simulink model "OSWEC_latching_force"  (R2021b)
settings: Solver=ode4  StartTime=0  StopTime=400  FixedStep=0.01  MaxStep=0.01  RelTol=1e-3  EnableMultiTasking=on
values from neighbouring files (symbols this model uses):
  simu = simulationClass()    [wecSimInputFile.m]
  waves = waveClass('regular')    [wecSimInputFile.m]
undefined symbols (not defined in the file or in its folder): body, constraint, geometry, hydroData, pto, X, Y, Z
libraries: nesl_utility x31, sm_lib x23, WECSim_Lib_Body_Elements x7, WECSim_Lib_Constraints x1, vrlib x1, WECSim_Lib_Frames x1
(part 3 of 3)

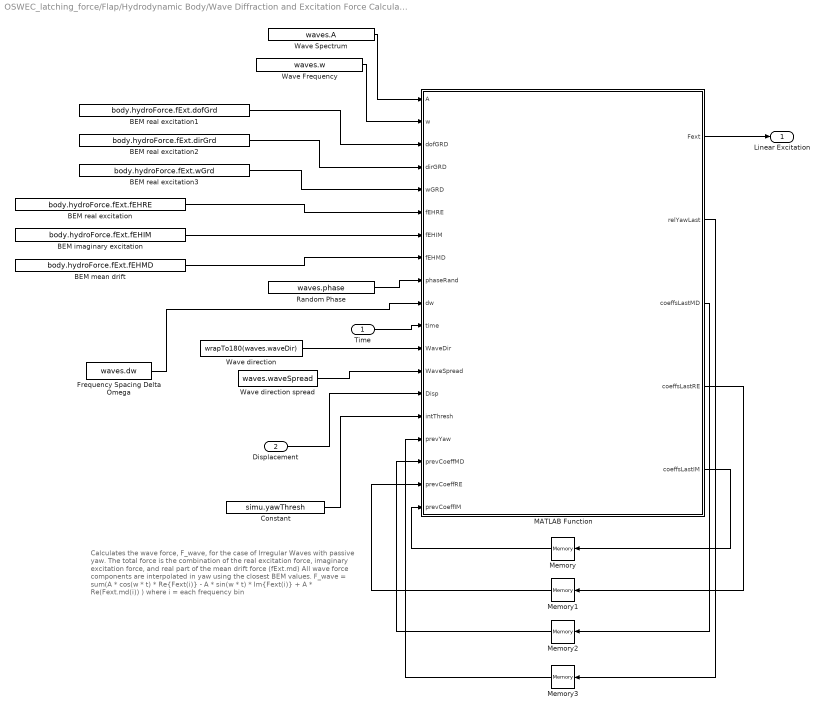
== system OSWEC_latching_force/Flap/Hydrodynamic Body/Wave Diffraction and Excitation Force Calculation/Linear Wave Excitation Force Variant Subsystem/Irregular Wave NonLinearYaw ==
  note: Calculates the wave force, F_wave, for the case of Irregular Waves with passive yaw.
      |
      | The total force is the combination of the real excitation force, imaginary excitation force, and real part of the mean drift force (fExt.md)
      |
      | All wave force components are interpolated in yaw using the closest BEM values.
      |
      | F_wave =   sum(A * cos(w * t) * Re{Fext(i)}
      |                            -  A * sin(w * t) * Im{Fext(i)}
      |                            + A * Re(Fext.md(i))
      |                            )
      |
      | where i = each frequency bin
  Time : Inport
  Displacement : Inport  Port=2
  BEM imaginary excitation : Constant  Value=body.hydroForce.fExt.fEHIM  VectorParams1D=off
  BEM mean drift : Constant  Value=body.hydroForce.fExt.fEHMD  VectorParams1D=off
  BEM real excitation : Constant  Value=body.hydroForce.fExt.fEHRE  VectorParams1D=off
  BEM real excitation1 : Constant  Value=body.hydroForce.fExt.dofGrd  VectorParams1D=off
  BEM real excitation2 : Constant  Value=body.hydroForce.fExt.dirGrd  VectorParams1D=off
  BEM real excitation3 : Constant  Value=body.hydroForce.fExt.wGrd  VectorParams1D=off
  Constant : Constant  Value=simu.yawThresh
  Frequency Spacing Delta Omega : Constant  Value=waves.dw  VectorParams1D=off
  MATLAB Function : MATLAB Function  TreatAsAtomicUnit=on
  Memory{,1..3} (4 alike) : Memory  InheritSampleTime=on  LinearizeAsDelay=on
  Random Phase : Constant  Value=waves.phase  VectorParams1D=off
  Wave Frequency : Constant  Value=waves.w  VectorParams1D=off
  Wave Spectrum : Constant  Value=waves.A  VectorParams1D=off
  Wave direction : Constant  Value=wrapTo180(waves.waveDir)  VectorParams1D=off
  Wave direction spread : Constant  Value=waves.waveSpread  VectorParams1D=off
  Linear Excitation : Outport
  wires:
  Displacement/1 -> MATLAB Function/14(Disp)
  Time/1 -> MATLAB Function/11(time)
  Wave direction spread/1 -> MATLAB Function/13(WaveSpread)
  BEM mean drift/1 -> MATLAB Function/8(fEHMD)
  Wave Spectrum/1 -> MATLAB Function/1(A)
  BEM real excitation1/1 -> MATLAB Function/3(dofGRD)
  Wave Frequency/1 -> MATLAB Function/2(w)
  Random Phase/1 -> MATLAB Function/9(phaseRand)
  Memory/1 -> MATLAB Function/19(prevCoeffIM)
  BEM real excitation/1 -> MATLAB Function/6(fEHRE)
  MATLAB Function/3(coeffsLastMD) -> Memory2/1
  Constant/1 -> MATLAB Function/15(intThresh)
  BEM imaginary excitation/1 -> MATLAB Function/7(fEHIM)
  Memory3/1 -> MATLAB Function/16(prevYaw)
  MATLAB Function/5(coeffsLastIM) -> Memory/1
  Wave direction/1 -> MATLAB Function/12(WaveDir)
  Frequency Spacing Delta Omega/1 -> MATLAB Function/10(dw)
  BEM real excitation2/1 -> MATLAB Function/4(dirGRD)
  BEM real excitation3/1 -> MATLAB Function/5(wGRD)
  Memory2/1 -> MATLAB Function/17(prevCoeffMD)
  MATLAB Function/2(relYawLast) -> Memory3/1
  MATLAB Function/4(coeffsLastRE) -> Memory1/1
  Memory1/1 -> MATLAB Function/18(prevCoeffRE)
  MATLAB Function/1(Fext) -> Linear Excitation/1

== system OSWEC_latching_force/Flap/Hydrodynamic Body/Wave Diffraction and Excitation Force Calculation/Linear Wave Excitation Force Variant Subsystem/No Wave Excitation Force ==
  Constant : Constant  Value=zeros(1,body.dof)
  Linear Excitation : Outport
  wires:
  Constant/1 -> Linear Excitation/1

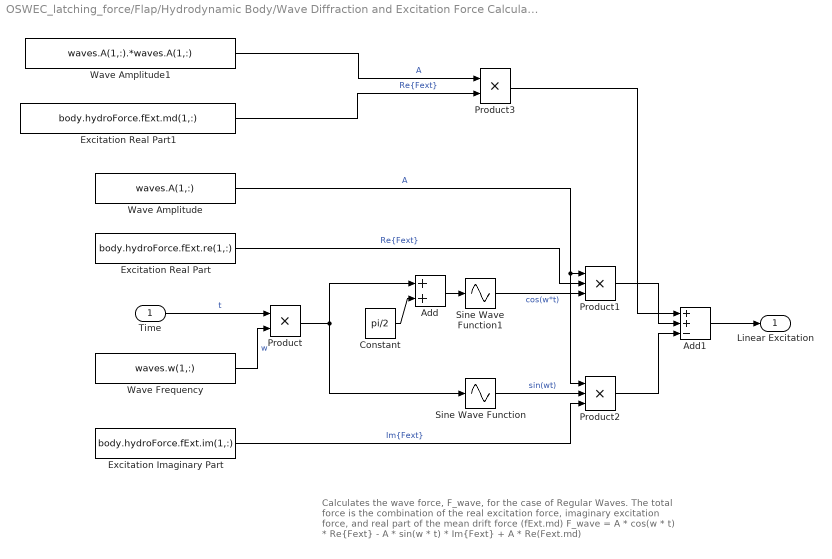
== system OSWEC_latching_force/Flap/Hydrodynamic Body/Wave Diffraction and Excitation Force Calculation/Linear Wave Excitation Force Variant Subsystem/Regular Wave Excitation Force ==
  note: Calculates the wave force, F_wave, for the case of Regular Waves.
      |
      | The total force is the combination of the real excitation force, imaginary excitation force, and real part of the mean drift force (fExt.md)
      |
      | F_wave =   A * cos(w * t) * Re{Fext}
      |                -  A * sin(w * t) * Im{Fext}
      |                + A * Re(Fext.md)
  Time : Inport
  Add : Sum
  Add1 : Sum  Inputs=++-
  Constant : Constant  Value=pi/2
  Excitation Imaginary Part : Constant  Value=body.hydroForce.fExt.im(1,:)  VectorParams1D=off
  Excitation Real Part : Constant  Value=body.hydroForce.fExt.re(1,:)  VectorParams1D=off
  Excitation Real Part1 : Constant  Value=body.hydroForce.fExt.md(1,:)  VectorParams1D=off
  Product : Product
  Product1 : Product  Inputs=3
  Product2 : Product  Inputs=3
  Product3 : Product
  Sine Wave Function : Sin  TimeSource=Use external signal  SampleTime=0
  Sine Wave Function1 : Sin  TimeSource=Use external signal  SampleTime=0
  Wave Amplitude : Constant  Value=waves.A(1,:)
  Wave Amplitude1 : Constant  Value=waves.A(1,:).*waves.A(1,:)
  Wave Frequency : Constant  Value=waves.w(1,:)
  Linear Excitation : Outport
  wires:
  Product3/1 -> Add1/1
  Excitation Real Part1/1 -> Product3/2  "Re{Fext}"
  Wave Amplitude1/1 -> Product3/1  "A"
  Constant/1 -> Add/2
  Add/1 -> Sine Wave Function1/1
  Wave Amplitude/1 -> Product1/1, Product2/1  "A"
  Add1/1 -> Linear Excitation/1
  Product2/1 -> Add1/3
  Product1/1 -> Add1/2
  Excitation Real Part/1 -> Product1/2  "Re{Fext}"
  Excitation Imaginary Part/1 -> Product2/3  "Im{Fext}"
  Sine Wave Function/1 -> Product2/2  "sin(wt)"
  Sine Wave Function1/1 -> Product1/3  "cos(w*t)"
  Product/1 -> Add/1, Sine Wave Function/1
  Wave Frequency/1 -> Product/2  "w"
  Time/1 -> Product/1  "t"

== system OSWEC_latching_force/Flap/Hydrodynamic Body/Wave Diffraction and Excitation Force Calculation/Linear Wave Excitation Force Variant Subsystem/Regular Wave NonLinear Yaw ==
  note: Calculates the wave force, F_wave, for the case of Regular Waves with passive yaw.
      |
      | The total force is the combination of the real excitation force, imaginary excitation force, and real part of the mean drift force (fExt.md)
      |
      | All wave force components are interpolated in yaw using the closest BEM values.
      |
      | F_wave =   A * cos(w * t) * Re{Fext}
      |                -  A * sin(w * t) * Im{Fext}
      |                + A * Re(Fext.md)
  Time : Inport
  Displacement : Inport  Port=2
  BEM imaginary excitation : Constant  Value=body.hydroForce.fExt.fEHIM  VectorParams1D=off
  BEM imaginary excitation1 : Constant  Value=body.hydroForce.fExt.dirGrd  VectorParams1D=off
  BEM mean drift : Constant  Value=body.hydroForce.fExt.fEHMD  VectorParams1D=off
  BEM real excitation : Constant  Value=body.hydroForce.fExt.fEHRE  VectorParams1D=off
  BEM real excitation1 : Constant  Value=body.hydroForce.fExt.dofGrd  VectorParams1D=off
  Constant : Constant  Value=simu.yawThresh
  MATLAB Function1 : MATLAB Function  TreatAsAtomicUnit=on
  Memory{,1..3} (4 alike) : Memory  InheritSampleTime=on  LinearizeAsDelay=on
  Wave Amplitude : Constant  Value=waves.A(1,:)
  Wave Frequency : Constant  Value=waves.w(1,:)
  Wave direction : Constant  Value=wrapTo180(waves.waveDir)  VectorParams1D=off
  Linear Excitation : Outport
  wires:
  Displacement/1 -> MATLAB Function1/10(Disp)
  Time/1 -> MATLAB Function1/8(time)
  MATLAB Function1/1(Fext) -> Linear Excitation/1
  Wave Frequency/1 -> MATLAB Function1/2(w)  "w"
  MATLAB Function1/5(coeffsLastIM) -> Memory/1
  MATLAB Function1/2(relYawLast) -> Memory3/1
  MATLAB Function1/4(coeffsLastRE) -> Memory1/1
  Memory3/1 -> MATLAB Function1/12(prevYaw)
  BEM mean drift/1 -> MATLAB Function1/7(fEHMD)
  Memory/1 -> MATLAB Function1/15(prevCoeffIM)
  Wave Amplitude/1 -> MATLAB Function1/1(A)  "A"
  MATLAB Function1/3(coeffsLastMD) -> Memory2/1
  BEM real excitation/1 -> MATLAB Function1/5(fEHRE)
  Wave direction/1 -> MATLAB Function1/9(WaveDir)
  BEM imaginary excitation/1 -> MATLAB Function1/6(fEHIM)
  BEM real excitation1/1 -> MATLAB Function1/3(dofGRD)
  Memory1/1 -> MATLAB Function1/14(prevCoeffRE)
  BEM imaginary excitation1/1 -> MATLAB Function1/4(dirGRD)
  Constant/1 -> MATLAB Function1/11(intThresh)
  Memory2/1 -> MATLAB Function1/13(prevCoeffMD)

== system OSWEC_latching_force/Flap/Hydrodynamic Body/Wave Diffraction and Excitation Force Calculation/Linear Wave Excitation Force Variant Subsystem/User Defined Wave Excitation Force ==
  note: Calculates the wave force, F_wave, for the case of User Defined Waves.
      |
      | F_wave = convolution calculation [1x6]
  InputWaveForceTimeHistory : FromWorkspace  VariableName=[waves.waveAmpTime(:,1),body.hydroForce.userDefinedFe]
  Linear Excitation : Outport
  wires:
  InputWaveForceTimeHistory/1 -> Linear Excitation/1

== system OSWEC_latching_force/Flap/Hydrodynamic Body/Wave Diffraction and Excitation Force Calculation/Nonlinear FK Force Variant Subsystem/No Nonlinear FroudeKrylov Force ==
  Constant : Constant  Value=zeros(1,body.dof)
  Nonlinear Excitation : Outport
  wires:
  Constant/1 -> Nonlinear Excitation/1

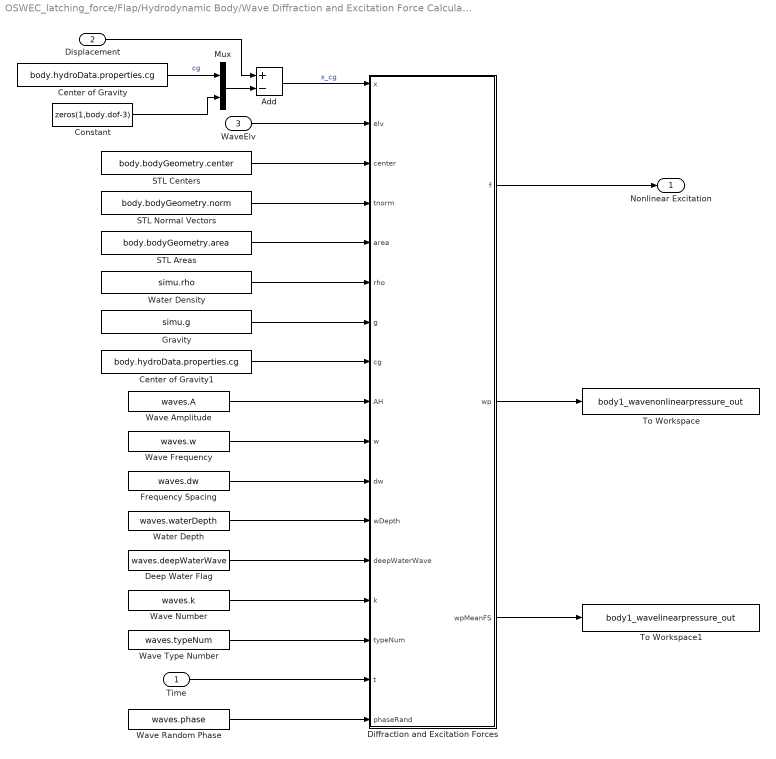
== system OSWEC_latching_force/Flap/Hydrodynamic Body/Wave Diffraction and Excitation Force Calculation/Nonlinear FK Force Variant Subsystem/With Nonlinear FroudeKrylov Force ==
  Time : Inport
  Displacement : Inport  Port=2
  WaveElv : Inport  Port=3
  Add : Sum  Inputs=+-
  Center of Gravity : Constant  Value=body.hydroData.properties.cg
  Center of Gravity1 : Constant  Value=body.hydroData.properties.cg
  Constant : Constant  Value=zeros(1,body.dof-3)
  Deep Water Flag : Constant  Value=waves.deepWaterWave
  Diffraction and Excitation Forces : MATLAB Function  TreatAsAtomicUnit=on
  Frequency Spacing : Constant  Value=waves.dw
  Gravity : Constant  Value=simu.g
  Mux : Mux  Inputs=2
  STL Areas : Constant  Value=body.bodyGeometry.area
  STL Centers : Constant  Value=body.bodyGeometry.center
  STL Normal Vectors : Constant  Value=body.bodyGeometry.norm
  To Workspace : ToWorkspace  VariableName=body1_wavenonlinearpressure_out  SaveFormat=Structure With Time  SampleTime=-1
      settings: Decimation=round(simu.dtOut/simu.dt,0)
  To Workspace1 : ToWorkspace  VariableName=body1_wavelinearpressure_out  SaveFormat=Structure With Time  SampleTime=-1
      settings: Decimation=round(simu.dtOut/simu.dt,0)
  Water Density : Constant  Value=simu.rho
  Water Depth : Constant  Value=waves.waterDepth
  Wave Amplitude : Constant  Value=waves.A
  Wave Frequency : Constant  Value=waves.w
  Wave Number : Constant  Value=waves.k
  Wave Random Phase : Constant  Value=waves.phase
  Wave Type Number : Constant  Value=waves.typeNum
  Nonlinear Excitation : Outport
  wires:
  STL Areas/1 -> Diffraction and Excitation Forces/5(area)
  Diffraction and Excitation Forces/2(wp) -> To Workspace/1
  Diffraction and Excitation Forces/3(wpMeanFS) -> To Workspace1/1
  Displacement/1 -> Add/1
  Constant/1 -> Mux/2
  Center of Gravity/1 -> Mux/1  "cg"
  Mux/1 -> Add/2
  Add/1 -> Diffraction and Excitation Forces/1(x)  "x_cg"
  Deep Water Flag/1 -> Diffraction and Excitation Forces/13(deepWaterWave)
  Wave Random Phase/1 -> Diffraction and Excitation Forces/17(phaseRand)
  Water Depth/1 -> Diffraction and Excitation Forces/12(wDepth)
  Wave Number/1 -> Diffraction and Excitation Forces/14(k)
  Wave Type Number/1 -> Diffraction and Excitation Forces/15(typeNum)
  Frequency Spacing/1 -> Diffraction and Excitation Forces/11(dw)
  Wave Frequency/1 -> Diffraction and Excitation Forces/10(w)
  Wave Amplitude/1 -> Diffraction and Excitation Forces/9(AH)
  Time/1 -> Diffraction and Excitation Forces/16(t)
  WaveElv/1 -> Diffraction and Excitation Forces/2(elv)
  STL Centers/1 -> Diffraction and Excitation Forces/3(center)
  STL Normal Vectors/1 -> Diffraction and Excitation Forces/4(tnorm)
  Water Density/1 -> Diffraction and Excitation Forces/6(rho)
  Gravity/1 -> Diffraction and Excitation Forces/7(g)
  Diffraction and Excitation Forces/1(f) -> Nonlinear Excitation/1
  Center of Gravity1/1 -> Diffraction and Excitation Forces/8(cg)

== system OSWEC_latching_force/Flap/Hydrodynamic Body/Wave Radiation Forces Calculation/SS CI and Constant-Damping-CoeVariant Subsystem/Constant Coefficients ==
  note: F = damping * velocity
  velocity : Inport
  Product : Product  Multiplication=Matrix(*)
  Radiation Damping Matrix : Constant  Value=body.hydroForce.fDamping
  Out1 : Outport
  wires:
  velocity/1 -> Product/2
  Product/1 -> Out1/1  "F_Single Frequency"
  Radiation Damping Matrix/1 -> Product/1

== system OSWEC_latching_force/Flap/Hydrodynamic Body/Wave Radiation Forces Calculation/SS CI and Constant-Damping-CoeVariant Subsystem/Convolution Integral Calculation ==
  note: Calculate the convolution integral using the radiation IRF (body.hydroForce.irkb) and the velocity.
  velocity : Inport
  CTTime : Constant  Value=simu.CTTime
  IRBK : Constant  Value=body.hydroForce.irkb
  MATLAB Function1 : MATLAB Function  TreatAsAtomicUnit=on  SystemSampleTime=simu.CTTime(2)-simu.CTTime(1)
  Rate Transition : RateTransition
  Reshape : Reshape
  Out1 : Outport
  wires:
  velocity/1 -> MATLAB Function1/1(velocity)
  CTTime/1 -> MATLAB Function1/3(CTTime)
  IRBK/1 -> MATLAB Function1/2(IRKB)
  MATLAB Function1/1(F_FM) -> Rate Transition/1
  Rate Transition/1 -> Reshape/1
  Reshape/1 -> Out1/1

== system OSWEC_latching_force/Flap/Hydrodynamic Body/Wave Radiation Forces Calculation/SS CI and Constant-Damping-CoeVariant Subsystem/State-Space Calculation  ==
  note: Calculate the radiation damping based on the state space formulation. Coefficients are defined in body.hydroForce.ssRadf
  velocity : Inport
  State-Space : StateSpace  A=body.hydroForce.ssRadf.A  B=body.hydroForce.ssRadf.B  C=body.hydroForce.ssRadf.C  D=body.hydroForce.ssRadf.D  InitialCondition=0
  Out1 : Outport
  wires:
  State-Space/1 -> Out1/1
  velocity/1 -> State-Space/1  "x"

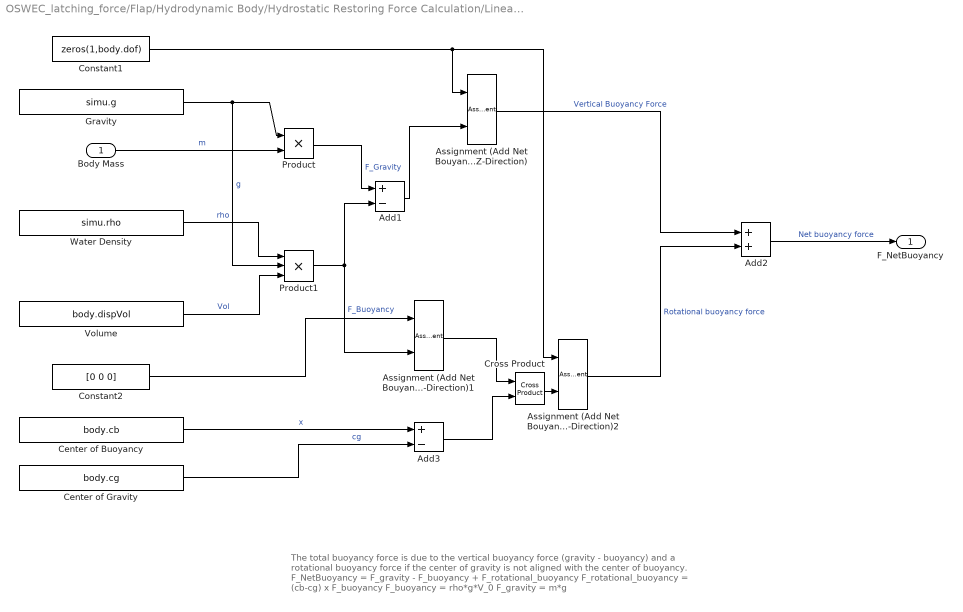
== system OSWEC_latching_force/Flap/Hydrodynamic Body/Hydrostatic Restoring Force Calculation/Linear and Nonlinear Restoring Force Variant Subsystem/Linear Hydrostatic Restoring Force/Net Buoyancy Force ==
  note: The total buoyancy force is due to the vertical buoyancy force (gravity - buoyancy) and a rotational buoyancy force if the center of gravity is not aligned with the center of buoyancy.
      |
      | F_NetBuoyancy = F_gravity - F_buoyancy + F_rotational_buoyancy
      |
      | F_rotational_buoyancy = (cb-cg) x F_buoyancy
      | F_buoyancy = rho*g*V_0
      | F_gravity = m*g
  Body Mass : Inport
  Add1 : Sum  Inputs=+-
  Add2 : Sum
  Add3 : Sum  Inputs=+-
  Assignment (Add Net Bouyancy Force to Z-Direction) : Assignment  IndexOptions=Index vector (dialog)  Indices=3  OutputSizes=1
  Assignment (Add Net Bouyancy Force to Z-Direction)1 : Assignment  IndexOptions=Index vector (dialog)  Indices=3  OutputSizes=1
  Assignment (Add Net Bouyancy Force to Z-Direction)2 : Assignment  IndexOptions=Index vector (dialog)  Indices=4:6  OutputSizes=1
  Center of Buoyancy : Constant  Value=body.cb
  Center of Gravity : Constant  Value=body.cg
  Constant1 : Constant  Value=zeros(1,body.dof)
  Constant2 : Constant  Value=[0 0 0]
  Cross Product : vrlib/Utilities/Cross Product
  Gravity : Constant  Value=simu.g
  Product : Product
  Product1 : Product  Inputs=3
  Volume : Constant  Value=body.dispVol
  Water Density : Constant  Value=simu.rho
  F_NetBuoyancy : Outport
  wires:
  Add1/1 -> Assignment (Add Net Bouyancy Force to Z-Direction)/2
  Body Mass/1 -> Product/2  "m"
  Cross Product/1 -> Assignment (Add Net Bouyancy Force to Z-Direction)2/2
  Add2/1 -> F_NetBuoyancy/1  "Net buoyancy force"
  Add3/1 -> Cross Product/2
  Constant2/1 -> Assignment (Add Net Bouyancy Force to Z-Direction)1/1
  Center of Gravity/1 -> Add3/2  "cg"
  Constant1/1 -> Assignment (Add Net Bouyancy Force to Z-Direction)/1, Assignment (Add Net Bouyancy Force to Z-Direction)2/1
  Center of Buoyancy/1 -> Add3/1  "x"
  Assignment (Add Net Bouyancy Force to Z-Direction)1/1 -> Cross Product/1
  Volume/1 -> Product1/3  "Vol"
  Assignment (Add Net Bouyancy Force to Z-Direction)/1 -> Add2/1  "Vertical Buoyancy Force"
  Water Density/1 -> Product1/1  "rho"
  Gravity/1 -> Product/1, Product1/2  "g"
  Product1/1 -> Assignment (Add Net Bouyancy Force to Z-Direction)1/2, Add1/2  "F_Buoyancy"
  Product/1 -> Add1/1  "F_Gravity"
  Assignment (Add Net Bouyancy Force to Z-Direction)2/1 -> Add2/2  "Rotational buoyancy force"

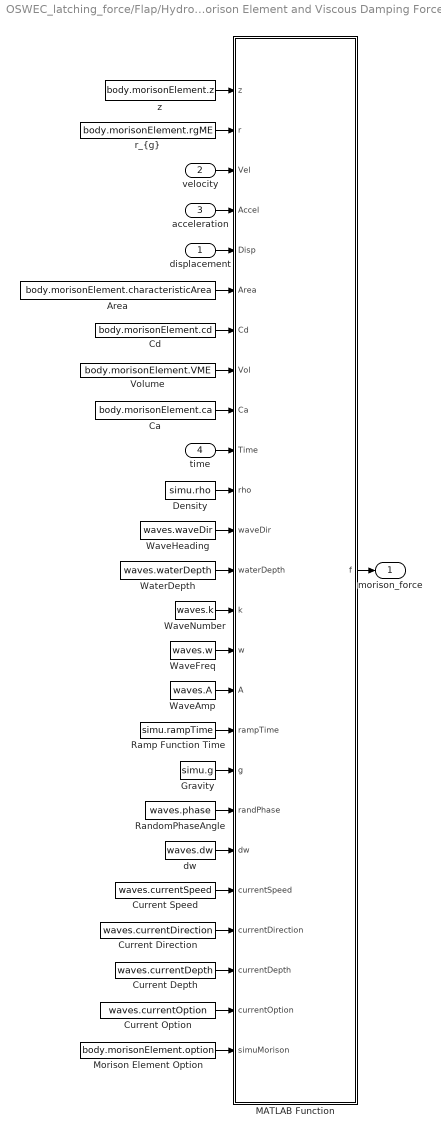
== system OSWEC_latching_force/Flap/Hydrodynamic Body/Morison Element and Viscous Damping Force Calculation/Morison Element Variant Subsystem/Morison Element On/Irregular Wave Morison Force ==
  displacement : Inport
  velocity : Inport  Port=2
  acceleration : Inport  Port=3
  time : Inport  Port=4
  Area : Constant  Value=body.morisonElement.characteristicArea  VectorParams1D=off
  Ca : Constant  Value=body.morisonElement.ca  VectorParams1D=off
  Cd : Constant  Value=body.morisonElement.cd  VectorParams1D=off
  Current Depth : Constant  Value=waves.currentDepth
  Current Direction : Constant  Value=waves.currentDirection
  Current Option : Constant  Value=waves.currentOption
  Current Speed : Constant  Value=waves.currentSpeed
  Density : Constant  Value=simu.rho
  Gravity : Constant  Value=simu.g
  MATLAB Function : MATLAB Function  TreatAsAtomicUnit=on
  Morison Element Option : Constant  Value=body.morisonElement.option
  Ramp Function Time : Constant  Value=simu.rampTime
  RandomPhaseAngle : Constant  Value=waves.phase  VectorParams1D=off
  Volume : Constant  Value=body.morisonElement.VME  VectorParams1D=off
  WaterDepth : Constant  Value=waves.waterDepth
  WaveAmp : Constant  Value=waves.A
  WaveFreq : Constant  Value=waves.w
  WaveHeading : Constant  Value=waves.waveDir
  WaveNumber : Constant  Value=waves.k
  dw : Constant  Value=waves.dw  VectorParams1D=off
  "r_{g}" : Constant  Value=body.morisonElement.rgME  VectorParams1D=off
  z : Constant  Value=body.morisonElement.z  VectorParams1D=off
  morison_force : Outport
  wires:
  Morison Element Option/1 -> MATLAB Function/25(simuMorison)
  Current Option/1 -> MATLAB Function/24(currentOption)
  Current Depth/1 -> MATLAB Function/23(currentDepth)
  Current Direction/1 -> MATLAB Function/22(currentDirection)
  Current Speed/1 -> MATLAB Function/21(currentSpeed)
  dw/1 -> MATLAB Function/20(dw)
  RandomPhaseAngle/1 -> MATLAB Function/19(randPhase)
  Gravity/1 -> MATLAB Function/18(g)
  Ramp Function Time/1 -> MATLAB Function/17(rampTime)
  WaveAmp/1 -> MATLAB Function/16(A)
  WaveFreq/1 -> MATLAB Function/15(w)
  WaveNumber/1 -> MATLAB Function/14(k)
  WaterDepth/1 -> MATLAB Function/13(waterDepth)
  WaveHeading/1 -> MATLAB Function/12(waveDir)
  Density/1 -> MATLAB Function/11(rho)
  time/1 -> MATLAB Function/10(Time)
  Ca/1 -> MATLAB Function/9(Ca)
  Volume/1 -> MATLAB Function/8(Vol)
  Cd/1 -> MATLAB Function/7(Cd)
  Area/1 -> MATLAB Function/6(Area)
  displacement/1 -> MATLAB Function/5(Disp)
  acceleration/1 -> MATLAB Function/4(Accel)
  velocity/1 -> MATLAB Function/3(Vel)
  "r_{g}"/1 -> MATLAB Function/2(r)
  z/1 -> MATLAB Function/1(z)
  MATLAB Function/1(f) -> morison_force/1

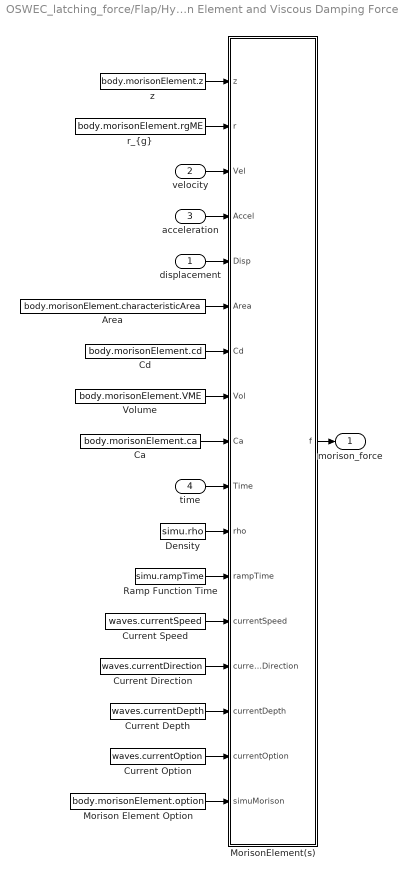
== system OSWEC_latching_force/Flap/Hydrodynamic Body/Morison Element and Viscous Damping Force Calculation/Morison Element Variant Subsystem/Morison Element On/No Wave Morison Force ==
  displacement : Inport
  velocity : Inport  Port=2
  acceleration : Inport  Port=3
  time : Inport  Port=4
  Area : Constant  Value=body.morisonElement.characteristicArea  VectorParams1D=off
  Ca : Constant  Value=body.morisonElement.ca  VectorParams1D=off
  Cd : Constant  Value=body.morisonElement.cd  VectorParams1D=off
  Current Depth : Constant  Value=waves.currentDepth
  Current Direction : Constant  Value=waves.currentDirection
  Current Option : Constant  Value=waves.currentOption
  Current Speed : Constant  Value=waves.currentSpeed
  Density : Constant  Value=simu.rho
  Morison Element Option : Constant  Value=body.morisonElement.option
  MorisonElement(s) : MATLAB Function  TreatAsAtomicUnit=on
  Ramp Function Time : Constant  Value=simu.rampTime
  Volume : Constant  Value=body.morisonElement.VME  VectorParams1D=off
  "r_{g}" : Constant  Value=body.morisonElement.rgME  VectorParams1D=off
  z : Constant  Value=body.morisonElement.z  VectorParams1D=off
  morison_force : Outport
  wires:
  Morison Element Option/1 -> MorisonElement(s)/17(simuMorison)
  Current Option/1 -> MorisonElement(s)/16(currentOption)
  Current Depth/1 -> MorisonElement(s)/15(currentDepth)
  Current Direction/1 -> MorisonElement(s)/14(currentDirection)
  Current Speed/1 -> MorisonElement(s)/13(currentSpeed)
  Ramp Function Time/1 -> MorisonElement(s)/12(rampTime)
  Density/1 -> MorisonElement(s)/11(rho)
  time/1 -> MorisonElement(s)/10(Time)
  Ca/1 -> MorisonElement(s)/9(Ca)
  Volume/1 -> MorisonElement(s)/8(Vol)
  Cd/1 -> MorisonElement(s)/7(Cd)
  Area/1 -> MorisonElement(s)/6(Area)
  displacement/1 -> MorisonElement(s)/5(Disp)
  acceleration/1 -> MorisonElement(s)/4(Accel)
  velocity/1 -> MorisonElement(s)/3(Vel)
  "r_{g}"/1 -> MorisonElement(s)/2(r)
  z/1 -> MorisonElement(s)/1(z)
  MorisonElement(s)/1(f) -> morison_force/1

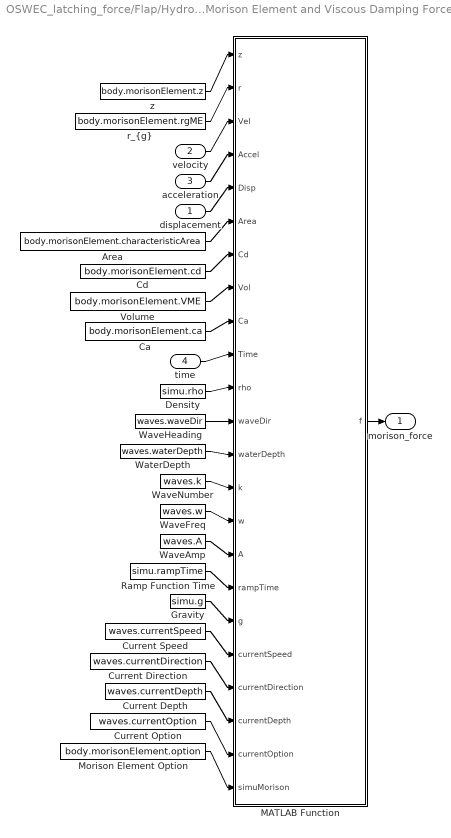
== system OSWEC_latching_force/Flap/Hydrodynamic Body/Morison Element and Viscous Damping Force Calculation/Morison Element Variant Subsystem/Morison Element On/Regular Wave Morison Force ==
  displacement : Inport
  velocity : Inport  Port=2
  acceleration : Inport  Port=3
  time : Inport  Port=4
  Area : Constant  Value=body.morisonElement.characteristicArea  VectorParams1D=off
  Ca : Constant  Value=body.morisonElement.ca  VectorParams1D=off
  Cd : Constant  Value=body.morisonElement.cd  VectorParams1D=off
  Current Depth : Constant  Value=waves.currentDepth
  Current Direction : Constant  Value=waves.currentDirection
  Current Option : Constant  Value=waves.currentOption
  Current Speed : Constant  Value=waves.currentSpeed
  Density : Constant  Value=simu.rho
  Gravity : Constant  Value=simu.g
  MATLAB Function : MATLAB Function  TreatAsAtomicUnit=on
  Morison Element Option : Constant  Value=body.morisonElement.option
  Ramp Function Time : Constant  Value=simu.rampTime
  Volume : Constant  Value=body.morisonElement.VME  VectorParams1D=off
  WaterDepth : Constant  Value=waves.waterDepth
  WaveAmp : Constant  Value=waves.A
  WaveFreq : Constant  Value=waves.w
  WaveHeading : Constant  Value=waves.waveDir
  WaveNumber : Constant  Value=waves.k
  "r_{g}" : Constant  Value=body.morisonElement.rgME  VectorParams1D=off
  z : Constant  Value=body.morisonElement.z  VectorParams1D=off
  morison_force : Outport
  wires:
  Current Speed/1 -> MATLAB Function/19(currentSpeed)
  WaveAmp/1 -> MATLAB Function/16(A)
  Gravity/1 -> MATLAB Function/18(g)
  WaveNumber/1 -> MATLAB Function/14(k)
  Ca/1 -> MATLAB Function/9(Ca)
  Current Direction/1 -> MATLAB Function/20(currentDirection)
  Area/1 -> MATLAB Function/6(Area)
  WaterDepth/1 -> MATLAB Function/13(waterDepth)
  acceleration/1 -> MATLAB Function/4(Accel)
  Density/1 -> MATLAB Function/11(rho)
  WaveHeading/1 -> MATLAB Function/12(waveDir)
  WaveFreq/1 -> MATLAB Function/15(w)
  Cd/1 -> MATLAB Function/7(Cd)
  displacement/1 -> MATLAB Function/5(Disp)
  Current Option/1 -> MATLAB Function/22(currentOption)
  Current Depth/1 -> MATLAB Function/21(currentDepth)
  time/1 -> MATLAB Function/10(Time)
  "r_{g}"/1 -> MATLAB Function/2(r)
  Ramp Function Time/1 -> MATLAB Function/17(rampTime)
  velocity/1 -> MATLAB Function/3(Vel)
  Volume/1 -> MATLAB Function/8(Vol)
  Morison Element Option/1 -> MATLAB Function/23(simuMorison)
  z/1 -> MATLAB Function/1(z)
  MATLAB Function/1(f) -> morison_force/1

== matlab function OSWEC_latching_force/Flap/Hydrodynamic Body/Morison Element and Viscous Damping Force Calculation/Morison Element Variant Subsystem/Morison Element On/No Wave Morison Force/MorisonElement(s) ==
  data: z input; f output; r input; Vel input; Accel input; Disp input; Area input; Cd input; Vol input; Ca input; Time input; rho input; rampTime input; currentSpeed input; currentDirection input; currentDepth input; currentOption input; simuMorison input
function f = noWaveMorison(z,r,Vel,Accel,Disp,Area,Cd,Vol,Ca,Time,rho,rampTime,currentSpeed,currentDirection,currentDepth,currentOption,simuMorison)

f = noWaveMorison(z,r,Vel,Accel,Disp,Area,Cd,Vol,Ca,Time,rho,rampTime,currentSpeed,currentDirection,currentDepth,currentOption,simuMorison);

end

== matlab function OSWEC_latching_force/Flap/Hydrodynamic Body/Morison Element and Viscous Damping Force Calculation/Morison Element Variant Subsystem/Morison Element On/Irregular Wave Morison Force/MATLAB Function ==
  data: z input; f output; r input; Vel input; Accel input; Disp input; Area input; Cd input; Vol input; Ca input; Time input; rho input; waveDir input; waterDepth input; k input; w input; A input; rampTime input; g input; randPhase input; dw input; currentSpeed input; currentDirection input; currentDepth input; currentOption input; simuMorison input
function f = irregWaveMorison(z,r,Vel,Accel,Disp,Area,Cd,Vol,Ca,Time,rho,waveDir,waterDepth,k,w,A,rampTime,g,randPhase,dw,currentSpeed,currentDirection,currentDepth,currentOption,simuMorison)

f = irregWaveMorison(z,r,Vel,Accel,Disp,Area,Cd,Vol,Ca,Time,rho,waveDir,waterDepth,k,w,A,rampTime,g,randPhase,dw,currentSpeed,currentDirection,currentDepth,currentOption,simuMorison);

end

== matlab function OSWEC_latching_force/Flap/Hydrodynamic Body/Nonlinear Wave Elevation/Linear or Instantaneous Free Surface/Instantaneous Water Free Surface/Instantaneous FS ==
  data: x input; center input; f output; cg input; AH input; w input; dw input; k input; typeNum input; t input; rampT input; phaseRand input; waveDir input
function f  = waveElevation(x,center,cg,AH,w,dw,k,typeNum,t,rampT,phaseRand,waveDir)

f  = waveElevation(x,center,cg,AH,w,dw,k,typeNum,t,rampT,phaseRand,waveDir);

end

== matlab function OSWEC_latching_force/Flap/Hydrodynamic Body/Structure/Motion Sensor/quaternion2EulXYZ ==
  data: Q input; E output
function E = quaternion2EulXYZ(Q)

E = quaternion2EulXYZ(Q);

end

== matlab function OSWEC_latching_force/Flap/Hydrodynamic Body/Wave Diffraction and Excitation Force Calculation/Linear Wave Excitation Force Variant Subsystem/Irregular Wave Excitation Force/MATLAB Function ==
  data: A input; Fext output; w input; fExtRE input; fExtIM input; phaseRand input; dw input; time input; WaveDir input; WaveSpread input; fExtMD input
function Fext = irregExcF(A,w,fExtRE,fExtIM,phaseRand,dw,time,WaveDir,WaveSpread,fExtMD)

Fext = irregExcF(A,w,fExtRE,fExtIM,phaseRand,dw,time,WaveDir,WaveSpread,fExtMD);

end

== matlab function OSWEC_latching_force/Flap/Hydrodynamic Body/Wave Diffraction and Excitation Force Calculation/Nonlinear FK Force Variant Subsystem/With Nonlinear FroudeKrylov Force/Diffraction and Excitation Forces ==
  data: x input; elv input; center input; f output; tnorm input; area input; rho input; g input; cg input; AH input; w input; dw input; wDepth input; deepWaterWave input; k input; typeNum input; t input; phaseRand input; wp output; wpMeanFS output
function [f, wp, wpMeanFS]  = nonFKForce(x,elv,center,tnorm,area,rho,g,cg,AH,w,dw,wDepth,deepWaterWave,k,typeNum,t,phaseRand)

[f, wp, wpMeanFS]  = nonFKForce(x,elv,center,tnorm,area,rho,g,cg,AH,w,dw,wDepth,deepWaterWave,k,typeNum,t,phaseRand);

end

== matlab function OSWEC_latching_force/Flap/Hydrodynamic Body/Wave Radiation Forces Calculation/SS CI and Constant-Damping-CoeVariant Subsystem/Convolution Integral Calculation/MATLAB Function1 ==
  data: velocity input; F_FM output; IRKB input; CTTime input
function F_FM = ConvolutionIntegral_interp(velocity, IRKB, CTTime)

F_FM = ConvolutionIntegral_interp(velocity, IRKB, CTTime);

end

== matlab function OSWEC_latching_force/Flap/Hydrodynamic Body/Yaw Force Transforms/Yaw Force Transforms ==
  data: yawNonLin input; F_Excitation output; dispGlobal input; F_RadiationDampingLocal input; F_AddedMassLocal input; F_ExcitationLocal input; F_RadiationDamping output; F_RestoringLocal input; F_AddedMass output; F_Restoring output
function [F_Excitation, F_RadiationDamping, F_AddedMass, F_Restoring] = fYawTransforms(yawNonLin, dispGlobal, F_RadiationDampingLocal, F_AddedMassLocal, F_ExcitationLocal, F_RestoringLocal)

[F_Excitation, F_RadiationDamping, F_AddedMass, F_Restoring] = fYawTransforms(yawNonLin, dispGlobal, F_RadiationDampingLocal, F_AddedMassLocal, F_ExcitationLocal, F_RestoringLocal);

end

== matlab function OSWEC_latching_force/Flap/Hydrodynamic Body/Wave Diffraction and Excitation Force Calculation/Linear Wave Excitation Force Variant Subsystem/Regular Wave NonLinear Yaw/MATLAB Function1 ==
  data: A input; w input; dofGRD input; dirGRD input; fEHRE input; fEHIM input; Fext output; fEHMD input; time input; WaveDir input; Disp input; intThresh input; prevYaw input; relYawLast output; prevCoeffMD input; prevCoeffRE input; prevCoeffIM input; coeffsLastMD output; coeffsLastRE output; coeffsLastIM output
function [Fext,relYawLast,coeffsLastMD,coeffsLastRE,coeffsLastIM] = regnLYaw(A,w,dofGRD,dirGRD,fEHRE,fEHIM, fEHMD,time,WaveDir,Disp, intThresh, prevYaw, prevCoeffMD, prevCoeffRE, prevCoeffIM)

%initialize outputs
Fext = zeros(1,6);
relYawLast=0;
coeffsLastMD=zeros(length(w),6); 
coeffsLastRE=zeros(length(w),6);
coeffsLastIM=zeros(length(w),6);

[Fext,relYawLast,coeffsLastMD,coeffsLastRE,coeffsLastIM] = regnLYaw(A,w,dofGRD,dirGRD,fEHRE,fEHIM, fEHMD,time,WaveDir,Disp, intThresh, prevYaw, prevCoeffMD, prevCoeffRE, prevCoeffIM);

end

== matlab function OSWEC_latching_force/Flap/Hydrodynamic Body/Yaw Kinematic Transforms/No B2B/Yaw Kinematic Transforms ==
  data: yawNonLin input; dispLoc output; dispGlobal input; velGlobal input; accGlobal input; velLoc output; accLoc output
function [dispLoc, velLoc, accLoc] = kinYawTransform(yawNonLin, dispGlobal, velGlobal, accGlobal)

[dispLoc, velLoc, accLoc] = kinYawTransformNoB2B(yawNonLin, dispGlobal, velGlobal, accGlobal);

end

== matlab function OSWEC_latching_force/Flap/Hydrodynamic Body/Yaw Kinematic Transforms/With B2B/Yaw Kinematic Transforms ==
  data: yawNonLin input; dispLoc output; dispGlobal input; velGlobal input; accGlobal input; velLoc output; accLoc output; numBody parameter
function [dispLoc, velLoc, accLoc] = kinYawTransformB2B(yawNonLin, dispGlobal, velGlobal, accGlobal, numBody)

[dispLoc, velLoc, accLoc] = kinYawTransformB2B(yawNonLin, dispGlobal, velGlobal, accGlobal, numBody);

end

== matlab function OSWEC_latching_force/Flap/Hydrodynamic Body/Morison Element and Viscous Damping Force Calculation/Morison Element Variant Subsystem/Morison Element On/Regular Wave Morison Force/MATLAB Function ==
  data: z input; f output; r input; Vel input; Accel input; Disp input; Area input; Cd input; Vol input; Ca input; Time input; rho input; waveDir input; waterDepth input; k input; w input; A input; rampTime input; g input; currentSpeed input; currentDirection input; currentDepth input; currentOption input; simuMorison input
function f = regWaveMorison(z,r,Vel,Accel,Disp,Area,Cd,Vol,Ca,Time,rho,waveDir,waterDepth,k,w,A,rampTime,g,currentSpeed,currentDirection,currentDepth,currentOption,simuMorison)

f = regWaveMorison(z,r,Vel,Accel,Disp,Area,Cd,Vol,Ca,Time,rho,waveDir,waterDepth,k,w,A,rampTime,g,currentSpeed,currentDirection,currentDepth,currentOption,simuMorison);

end

== matlab function OSWEC_latching_force/Flap/Hydrodynamic Body/Hydrostatic Restoring Force Calculation/Linear and Nonlinear Restoring Force Variant Subsystem/Nonlinear Hydrostatic Restoring Force/Restoring Forces ==
  data: x input; elv input; center input; f output; tnorm input; area input; rho input; g input; cg input; p output; mass input
function [f,p]  = nonLinearBuoyancy(x,elv,center,tnorm,area,rho,g,cg,mass)

[f,p]  = nonLinearBuoyancy(x,elv,center,tnorm,area,rho,g,cg,mass);

end

== matlab function OSWEC_latching_force/Subsystem/MATLAB Function ==
  data: vel input; Force output; tlatch input; tunlatch input; velprev input; T input; tlatch output; tunlatch output; vel output; H input; fe input; Fexc input
function [Force,tlatch,tunlatch,vel] = fcn(vel,tlatch,tunlatch,velprev,T,H,fe,Fexc)

if (diff(sign([vel,velprev]))~=0 && tlatch==0 && tunlatch>.5) || (tlatch>0 && abs(Fexc)<(H/(2))*fe*sin((pi/2)*(1-(5.6956/T))))
    Force = -2e8*vel;
    tlatch = tlatch + .01;
    tunlatch = 0;
else
    Force = 0;
    tunlatch = tunlatch+.01;
    tlatch = 0;
end
end

== matlab function OSWEC_latching_force/Flap/Hydrodynamic Body/Wave Diffraction and Excitation Force Calculation/Linear Wave Excitation Force Variant Subsystem/Irregular Wave NonLinearYaw/MATLAB Function ==
  data: A input; w input; dofGRD input; dirGRD input; wGRD input; fEHRE input; fEHIM input; Fext output; fEHMD input; phaseRand input; dw input; time input; WaveDir input; WaveSpread input; Disp input; intThresh input; prevYaw input; relYawLast output; prevCoeffMD input; prevCoeffRE input; prevCoeffIM input; coeffsLastMD output; coeffsLastRE output; coeffsLastIM output
function [Fext,relYawLast,coeffsLastMD,coeffsLastRE,coeffsLastIM] = irregnLYaw(A,w,dofGRD,dirGRD,wGRD,fEHRE,fEHIM, fEHMD, phaseRand,dw,time,WaveDir,WaveSpread, Disp, intThresh, prevYaw, prevCoeffMD, prevCoeffRE, prevCoeffIM)

%initialize outputs
Fext = zeros(1,6);
relYawLast=0;
coeffsLastMD=zeros(length(w),6);
coeffsLastRE=zeros(length(w),6);
coeffsLastIM=zeros(length(w),6);

[Fext,relYawLast,coeffsLastMD,coeffsLastRE,coeffsLastIM] = irregnLYaw(A,w,dofGRD,dirGRD,wGRD,fEHRE,fEHIM, fEHMD, phaseRand,dw,time,WaveDir,WaveSpread, Disp, intThresh, prevYaw, prevCoeffMD, prevCoeffRE, prevCoeffIM);

end
